simulink model "ysw6_1"  (R2014a)
settings: Solver=ode45  StartTime=0.0  StopTime=10  RelTol=1e-3
settings Model: Creator=Administrator  LastModifiedBy=Administrator

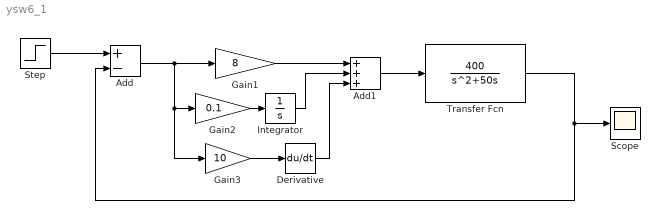
== system ysw6_1 ==
  Add : Sum  Inputs=+-
  Add1 : Sum  Inputs=+++
  Derivative : Derivative
  Gain1 : Gain  Gain=8
  Gain2 : Gain  Gain=0.1
  Gain3 : Gain  Gain=10
  Integrator : Integrator
  Scope : Scope
      settings: TimeRange=10  YMin=0  YMax=1.5e+25
  Step : Step  Time=0  SampleTime=0
  Transfer Fcn : TransferFcn  Numerator=[400]  Denominator=[1 50 0]
  wires:
  Step/1 -> Add/1
  Add1/1 -> Transfer Fcn/1
  Gain1/1 -> Add1/1
  Gain2/1 -> Integrator/1
  Integrator/1 -> Add1/2
  Gain3/1 -> Derivative/1
  Derivative/1 -> Add1/3
  Add/1 -> Gain3/1, Gain2/1, Gain1/1
  Transfer Fcn/1 -> Add/2, Scope/1
